simulink model "Todo_EKF_1er_Riccati"  (R2017b)
settings: Solver=FixedStepDiscrete  StartTime=0.0  StopTime=60  FixedStep=0.02  RelTol=1e-3  EnableMultiTasking=on
InitFcn:
  | load('Pose_integration_R_L.mat')
  | ProcNoiseD=0.01^2; % is a variance
  | ProcNoiseTheta=0.001^2; % is a variance
StopFcn:
  | I = imread('Enviroment.png');
  | x = [0 35.9];
  | y=[23.31 0];
  | image(I,'XData',x,'YData',y);
  | axis xy;
  | hold on
  | plot (Pose_est.Data(:,1), Pose_est.Data(:,2),'b');
  | plot (Pose_t.Data(:,1),Pose_t.Data(:,2),'r');
  | len=length(Pose_t.Data);
  | for i=1:round(len/15):len
  |     plot_ellipse(Pk.signals.values(1:2,1:2,i),[Pose_est.Data(i,1), Pose_est.Data(i,2)],'g');
  | end
settings Model: Creator=antonio  LastModifiedBy=DNI 53339557
settings DataIOCC: LimitDataPoints=on  SaveFormat=Array
settings OptimizationCC: LifeSpan=inf
settings DebuggingCC: UnderspecifiedInitializationDetection=Classic  MergeDetectMultiDrivingBlocksExec=none  SolverPrmCheckMsg=warning  StateNameClashWarn=warning  SFUnexpectedBacktrackingDiag=warning  SFNoUnconditionalDefaultTransitionDiag=warning  SFExecutionAtInitializationDiag=none
settings HardwareCC: ProdBitPerPointer=32  ProdBitPerSizeT=32  ProdBitPerPtrDiffT=32  ProdLargestAtomicFloat=None  ProdIntDivRoundTo=Undefined  ProdEndianess=Unspecified  ProdWordSize=32  ProdHWDeviceType=32-bit Generic
settings ModelReferenceCC: PropagateSignalLabelsOutOfModel=off
settings CodeAppCC: StateflowObjectComments=on
settings GRTTargetCC: TargetLangStandard=C89/C90 (ANSI)  GeneratePreprocessorConditionals=Disable all
settings ConfigComp: CovMetricSettings=dw  CovHtmlReporting=on  CovSaveCumulativeToWorkspaceVar=on  CovSaveSingleToWorkspaceVar=on  CovExternalEMLEnable=off

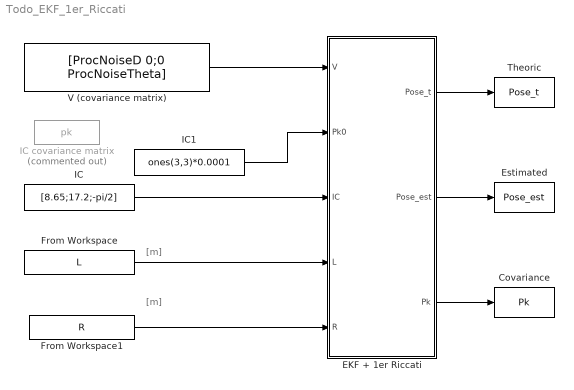
== system Todo_EKF_1er_Riccati ==
  note: [m]
  note: [m]
  Covariance : ToWorkspace  VariableName=Pk  SaveFormat=Structure With Time  SampleTime=-1
  EKF + 1er Riccati : MATLAB Function  TreatAsAtomicUnit=on
  Estimated : ToWorkspace  VariableName=Pose_est  SaveFormat=Timeseries  SampleTime=-1
  From Workspace : FromWorkspace  VariableName=L  SampleTime=0
  From Workspace1 : FromWorkspace  VariableName=R  SampleTime=0
  IC : Constant  Value=[8.65;17.2;-pi/2]
  IC covariance matrix : FromWorkspace  Commented=on  VariableName=pk
  IC1 : Constant  Value=ones(3,3)*0.0001
  Theoric : ToWorkspace  VariableName=Pose_t  SaveFormat=Timeseries  SampleTime=-1
  V (covariance matrix) : Constant  Value=[ProcNoiseD 0;0 ProcNoiseTheta]  VectorParams1D=off
  wires:
  IC/1 -> EKF + 1er Riccati/3(IC)
  EKF + 1er Riccati/1(Pose_t) -> Theoric/1
  EKF + 1er Riccati/2(Pose_est) -> Estimated/1
  From Workspace1/1 -> EKF + 1er Riccati/5(R)
  From Workspace/1 -> EKF + 1er Riccati/4(L)
  V (covariance matrix)/1 -> EKF + 1er Riccati/1(V)
  EKF + 1er Riccati/3(Pk) -> Covariance/1
  IC1/1 -> EKF + 1er Riccati/2(Pk0)

== matlab function Todo_EKF_1er_Riccati/EKF + 1er Riccati ==
  data: V input; Pk0 input; Pose_t output; Pose_est output; IC input; L input; R input; Pk output
function [Pose_t,Pose_est,Pk] = fcn(V,Pk0,IC,L,R) % IC->Initial Condition [xo,yo,th0]
                                   % R and L are the displacements of
                                   % wheels [m]
persistent x_w y_w suma_theta Pkp x_est x_t %  internal variable to be mantain its values

ts=0.02; % sample time

%%%%%%%%%%%%%%%%%%%%%%%%%%%%%%%%%%%%%%%%%%%%%%%%%%%%%%%%%%%%%%%%%%%%%%%%%%
% %%%%%%%%%%%%%%   Read Initial condition   %%%%%%%%%%%%%%%%%%%%%%%%%%%%%%
x_ini=IC(1);
y_ini=IC(2);
theta_ini=IC(3);
P_ini=Pk0;

%%%%%%%%%%%%%%%%%%%%%%%%%%%%%%%%%%%%%%%%%%%%%%%%%%%%%%%%%%%%%%%%%%%%%%%%%%
%%%%%%%%%%%%%%%   variable initialitation  %%%%%%%%%%%%%%%%%%%%%%%%%%%%%%
if isempty (x_w)
    x_w=x_ini;
    y_w=y_ini;
    suma_theta=theta_ini;
    Pkp=P_ini;
    x_est=[x_ini; y_ini; theta_ini];
    x_t=x_est;
end
%%%%%%%%%%%%%%%%%%%%%%%%%%%%%%%%%%%%%%%%%%%%%%%%%%%%%%%%%%%%%%%%%%%%%%%%%%
%%%%%%%%%%%%%%%%%  compute the odometry    %%%%%%%%%%%%%%%%%%%%%%%%%%%%%%%
delta_th=(R-L)/0.52;
delta_d=(R+L)/2;
%%%%%%%%%%%%%%%%%%%%%%%%%%%%%%%%%%%%%%%%%%%%%%%%%%%%%%%%%%%%%%%%%%%%%%%%%%
%%%%%%%%%%%%%%%%%  integration of the robot pose %%%%%%%%%%%%%%%%%%%%%%%%%%
x_w=x_w + delta_d*cos(suma_theta)+V(1,1);
y_w=y_w + delta_d*sin(suma_theta)+V(1,1);
suma_theta=mod(suma_theta+delta_th+V(2,2),2*pi);  
x_t=[x_w; y_w; suma_theta];
%%%%%%%%%%%%%%%%%%%%%%%%%%%%%%%%%%%%%%%%%%%%%%%%%%%%%%%%%%%%%%%%%%%%%%%%%%
%%%%%%%%%%%%%%%%%  Build the Jacocian %%%%%%%%%%%%%%%%%%%%%%%%%%%%%%%%%%%%
Fx=[1 0 -(delta_d*sin(suma_theta+delta_th));
    0 1 (delta_d*cos(suma_theta+delta_th));
    0 0 1];
Fv=[cos(suma_theta+delta_th) -(delta_d*sin(suma_theta+delta_th));
    sin(suma_theta+delta_th) (delta_d*cos(suma_theta+delta_th));
    0 1];
%%%%%%%%%%%%%%%%%%%%%%%%%%%%%%%%%%%%%%%%%%%%%%%%%%%%%%%%%%%%%%%%%%%%%%%%%%
%%%%%%%%%%%%%%%%% Compute the EKF Truncated Taylor %%%%%%%%%%%%%%%%%%%%%%%%
x_est=x_est+Fx*(x_t-x_est)+Fv*diag(V);
Pkp=Fx*Pkp*Fx'+Fv*V*Fv';
%%%%%%%%%%%%%%%%%%%%%%%%%%%%%%%%%%%%%%%%%%%%%%%%%%%%%%%%%%%%%%%%%%%%%%%%%%
%%%%%%%%%%%%%%%%%  output variable %%%%%%%%%%%%%%%%%%%%%%%%%%%%%%%%%%%%%%%

Pose_t=x_t;
Pose_est=x_est;
Pk=Pkp;

end
